simulink model "Lab4_Part6"  (R2023a)
settings: Solver=ode23tb  StartTime=0.0  StopTime=0.1  RelTol=1e-6  EnableMultiTasking=on
libraries: spsSeriesRLCBranchLib x4, spsCurrentMeasurementLib x1, spsDCVoltageSourceLib x1, spsDiodeLib x1, spsIdealSwitchLib x1, spsMosfetLib x1, simulink_need_slupdate x1, simulink x1, spsVoltageMeasurementLib x1, sps_lib x1
settings Model: Creator=dkozel  LastModifiedBy=swooradi
settings SolverCC: ZeroCrossAlgorithm=Adaptive  AlgebraicLoopSolver=TrustRegion  SolverResetMethod=Robust
settings DataIOCC: LimitDataPoints=on  SaveFormat=Array  ReturnWorkspaceOutputs=off
settings OptimizationCC: LifeSpan=inf
settings DebuggingCC: MaskedZcDiagnostic=none  IgnoredZcDiagnostic=none  UnconnectedInputMsg=warning  UnconnectedOutputMsg=warning  UnconnectedLineMsg=warning  SFUnexpectedBacktrackingDiag=warning  SFNoUnconditionalDefaultTransitionDiag=warning  SFExecutionAtInitializationDiag=none  ArithmeticOperatorsInVariantConditions=warning
settings HardwareCC: ProdBitPerPointer=32  ProdBitPerSizeT=32  ProdBitPerPtrDiffT=32  ProdLargestAtomicFloat=None  ProdIntDivRoundTo=Undefined  ProdEndianess=Unspecified  ProdWordSize=32  ProdHWDeviceType=32-bit Generic
settings ModelReferenceCC: EnableRefExpFcnMdlSchedulingChecks=on  PropagateSignalLabelsOutOfModel=off
settings SFSimCC: SimUseLocalCustomCode=off  CustomCodeUndefinedFunction=UseInterfaceOnly
settings RTWCC: RTWUseLocalCustomCode=off
settings CodeAppCC: StateflowObjectComments=on
settings GRTTargetCC: TargetLangStandard=C89/C90 (ANSI)
settings ConfigComp: CovMetricSettings=dw  CovSaveCumulativeToWorkspaceVar=on  CovSaveSingleToWorkspaceVar=on  CovExternalEMLEnable=off
settings SimscapeCC: SimscapeNormalizeSystem=off

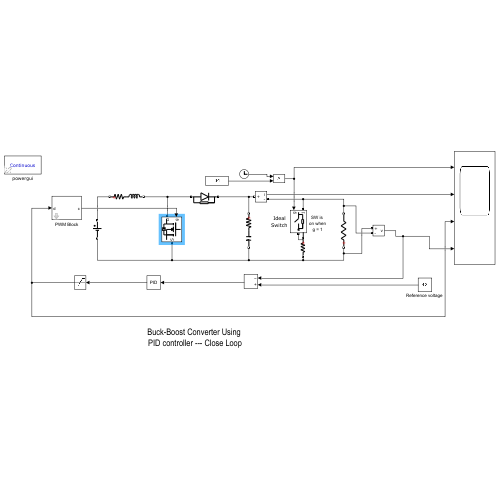
[thumbnail: Simulink's stored preview of the top-level diagram]
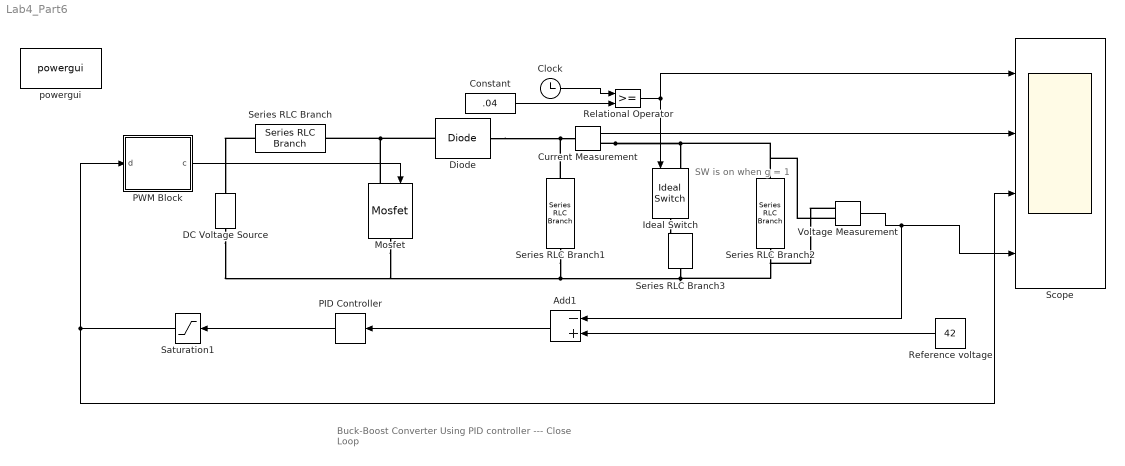
== system Lab4_Part6 ==
  note: Buck-Boost Converter Using
      | PID controller --- Close Loop
  note: SW is
      | on when
      | g = 1
  Add1 : Sum  Inputs=-+
  Clock : Clock
  Constant : Constant  Value=.04
  Current Measurement : spsCurrentMeasurementLib/Current Measurement  PhasorSimulation=off  OutputType=Complex  PSBequivalent=0
  DC Voltage Source : spsDCVoltageSourceLib/DC Voltage Source  Amplitude=14  Measurements=None
  Diode : spsDiodeLib/Diode  Ron=0.001  Lon=0  Vf=0.8  IC=0  UseSnubber=off  Rs=500  Cs=250e-9  Measurements=off
  Ideal Switch : spsIdealSwitchLib/Ideal Switch  Ron=0.001  Lon=0  IC=0  Rs=1e5  Cs=inf  Measurements=off
  Mosfet : spsMosfetLib/Mosfet  Ron=0.1  Lon=0  Rd=0.01  Vfd=0  IC=0  Rs=1e5  Cs=inf  Measurements=off
  PID Controller : simulink_need_slupdate/PID Controller  P=0.005  I=1  D=0
  PWM Block : Subsystem  mask{fs=200e3}
      mask prompts: fs "Switching fFrequency"
  "Reference voltage " : Constant  Value=42
  Relational Operator : RelationalOperator  OutDataTypeStr=boolean  InputSameDT=off
  Saturation1 : Saturate  UpperLimit=0.99  LowerLimit=0
  Scope : Scope  NumInputPorts=4
  Series RLC Branch : spsSeriesRLCBranchLib/Series RLC Branch  LConnTagsString=__new0  RConnTagsString=__new0  BranchType=RL  Resistance=0.08  Inductance=100e-6  SetiL0=off  InitialCurrent=0  Capacitance=1e-6  Setx0=off  InitialVoltage=0  Measurements=None
  Series RLC Branch1 : spsSeriesRLCBranchLib/Series RLC Branch  LConnTagsString=__new0  RConnTagsString=__new0  BranchType=RC  Resistance=0.1  Inductance=1e-3  SetiL0=off  InitialCurrent=0  Capacitance=697e-6  Setx0=on  InitialVoltage=0  Measurements=None
  Series RLC Branch2 : spsSeriesRLCBranchLib/Series RLC Branch  LConnTagsString=__new0  RConnTagsString=__new0  BranchType=R  Resistance=84  Inductance=1e-3  SetiL0=off  InitialCurrent=0  Capacitance=697e-6  Setx0=off  InitialVoltage=0  Measurements=None
  Series RLC Branch3 : spsSeriesRLCBranchLib/Series RLC Branch  LConnTagsString=__new0  RConnTagsString=__new0  BranchType=R  Resistance=84  Inductance=1e-3  SetiL0=off  InitialCurrent=0  Capacitance=1e-6  Setx0=off  InitialVoltage=0  Measurements=Branch voltage and current
  Voltage Measurement : spsVoltageMeasurementLib/Voltage Measurement  PhasorSimulation=off  OutputType=Complex  PSBequivalent=0
  powergui : sps_lib/powergui  Priority=1  SimulationMode=Continuous  SampleTime=1e-8  frequency=60  Iterations=50  frequencyindice=0  Pbase=100e6  ErrMax=1e-4  UnitsV=kV  UnitsW=MW  buscounter=0  FunctionMessages=off  echomessages=off  EnableUseOfTLC=off  CurrentSourceSwitches=on  DisableSnubberDevices=off  DisableRonSwitches=off  DisableVfSwitches=off  DisplayEquations=off  AutomaticDiscreteSolvers=off  SolverType=Tustin/Backward Euler (TBE)  Interpol=off  ExternalGateDelay=off  methode=off  Ts=0  x0status=blocks  SPID=off  SwTol=0  HookPort=off  NonlinearTolerance=1e-4  nMaxIteration=100  ContinueOnMaxIteration=off  RestoreLinks=warning  ResistiveCurrentMeasurement=off  Frange=[0:2:500]  Ylog=off  Xlog=on  ShowGrid=off  save=off  variable=ZData  structure=tpa14cfcc1_35b5_40eb_8b70_049b43167a68  ZoomFFT=off  StartTime=0.0  cycles=1  DisplayStyle=1  fundamental=60  FreqAxis=off  MaxFrequency=1000  frequencyindicesteady=1  RmsSteady=1  display=off
  wires:
  PWM Block/1(c) -> Mosfet/1
  Voltage Measurement/1 -> Add1/1, Scope/4
  Add1/1 -> PID Controller/1
  Constant/1 -> Relational Operator/2
  Clock/1 -> Relational Operator/1
  Relational Operator/1 -> Scope/1, Ideal Switch/1
  PID Controller/1 -> Saturation1/1
  Saturation1/1 -> Scope/3, PWM Block/1(d)
  Current Measurement/1 -> Scope/2
  "Reference voltage "/1 -> Add1/2
  connections:
  Series RLC Branch3/RConn1 -- Series RLC Branch2/LConn1 -- Voltage Measurement/LConn1 -- DC Voltage Source/LConn1 -- Mosfet/RConn1 -- Series RLC Branch1/RConn1
  Current Measurement/RConn1 -- Series RLC Branch2/RConn1 -- Voltage Measurement/LConn2 -- Ideal Switch/LConn1
  Series RLC Branch1/LConn1 -- Diode/RConn1 -- Current Measurement/LConn1
  Ideal Switch/RConn1 -- Series RLC Branch3/LConn1
  Mosfet/LConn1 -- Diode/LConn1 -- Series RLC Branch/RConn1
  Series RLC Branch/LConn1 -- DC Voltage Source/RConn1

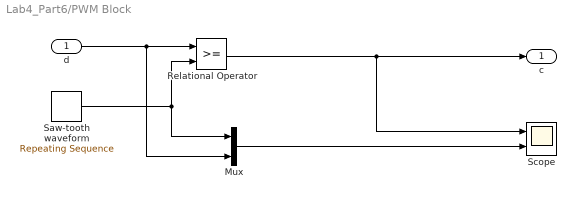
== system Lab4_Part6/PWM Block ==
  d : Inport
  Mux : Mux  Inputs=2
  Relational Operator : RelationalOperator  OutDataTypeStr=boolean  InputSameDT=off
  Saw-tooth waveform : simulink/Sources/Repeating Sequence  rep_seq_t=[0 1/fs]  rep_seq_y=[0 1]
  Scope : Scope  NumInputPorts=2
  c : Outport  VectorParamsAs1DForOutWhenUnconnected=off
  wires:
  d/1 -> Mux/2, Relational Operator/1
  Saw-tooth waveform/1 -> Mux/1, Relational Operator/2
  Relational Operator/1 -> c/1, Scope/1
  Mux/1 -> Scope/2
